simulink model "ProyectoAutomatasSimulink_jona"  (R2015a)
settings: Solver=ode45  SolverMode=SingleTasking  StartTime=0.0  StopTime=inf  FixedStep=dt
values from neighbouring files (symbols this model uses):
  yt0 = 45    [ProyectoAutomatas.m]
libraries: opclib x6, vrlib x1
settings Model: Creator=Garcia Obredor  LastModifiedBy=PIJON 2
settings DataIOCC: SignalLoggingSaveFormat=ModelDataLogs
settings OptimizationCC: BlockReduction=off  BooleanDataType=off  SimCompilerOptimization=on
settings DebuggingCC: SaveWithParameterizedLinksMsg=none  UnderspecifiedInitializationDetection=Classic  MergeDetectMultiDrivingBlocksExec=none  SignalResolutionControl=TryResolveAllWithWarning  MultiTaskDSMMsg=warning  MultiTaskCondExecSysMsg=none
settings HardwareCC: TargetBitPerPointer=64  TargetLongLongMode=on  TargetIntDivRoundTo=Zero  TargetEndianess=LittleEndian  TargetWordSize=64  TargetHWDeviceType=MATLAB Host  ProdEqTarget=off

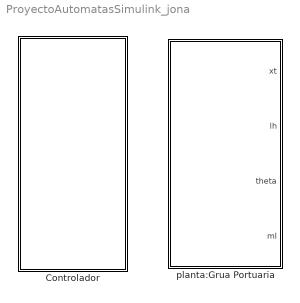
== system ProyectoAutomatasSimulink_jona ==
  Controlador : Subsystem
  planta:Grua Portuaria : Subsystem

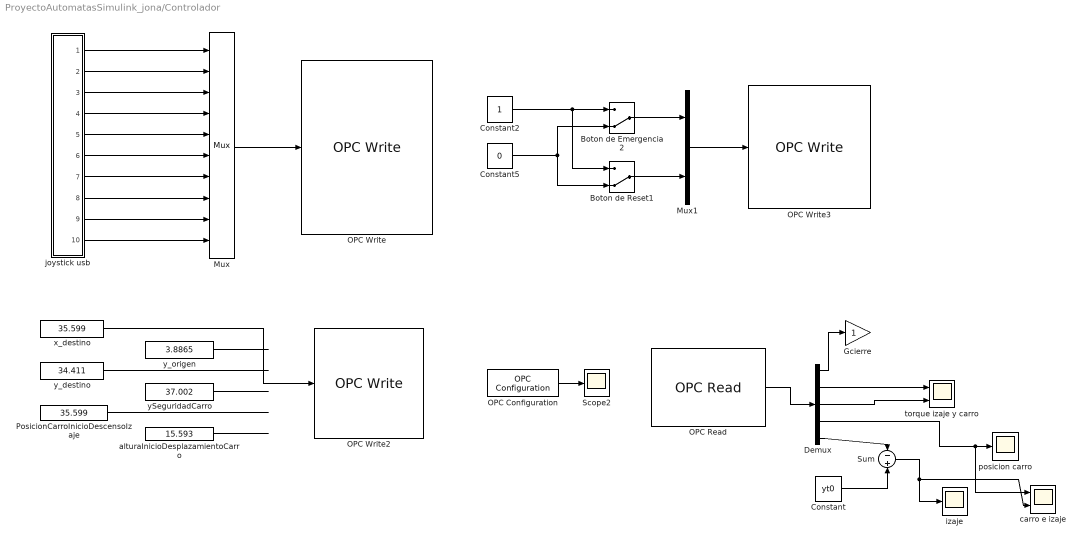
== system ProyectoAutomatasSimulink_jona/Controlador ==
  Boton de Emergencia2 : ManualSwitch  CurrentSetting=0
  Boton de Reset1 : ManualSwitch  CurrentSetting=0
  Constant : Constant  Value=yt0
  Constant2 : Constant
  Constant5 : Constant  Value=0
  Demux : Demux  Outputs=5
  Gcierre : Gain
  Mux : Mux  Inputs=10
  Mux1 : Mux  Inputs=2
  OPC Configuration : opclib/OPC Configuration  opcServers=localhost/CoDeSys.OPC.DA/10  errMissingItems=Error  errReadWrite=Warn  errShutdown=Error  errRTViolation=Warn  rtEnable=on  speedup=1  showLatency=on  beingUsed=on
  OPC Read : opclib/OPC Read  serverHost=localhost  serverID=CoDeSys.OPC.DA  itemIDs=PLC_GW3.Application.Global.Gcierre, PLC_GW3.Application.Global.Th, PLC_GW3.Application.Global.Tt, PLC_GW3.Application.Global.xt, PLC_GW3.Application.Global.lh  readMode=Synchronous (cache)  dataType=double  updateRate=0.001  showQual=off  showTS=off  tsMode=Seconds since start
  OPC Write : opclib/OPC Write  serverHost=localhost  serverID=CoDeSys.OPC.DA  itemIDs=PLC_GW3.Application.Global.BotonAbrirGancho, PLC_GW3.Application.Global.BotonCerrarGancho, PLC_GW3.Application.Global.BotonOperarMaq, PLC_GW3.Application.Global.BotonPararMaq, PLC_GW3.Application.Global.BotonModoAutomatico, PLC_GW3.Application.Global.BotonModoManual, PLC_GW3.Application.Global.PalancaCarro, PLC_GW3.Application.Global.PalancaIzaje, PLC_GW3.Application.Global.BotonActivaControlAngulo, PLC_GW3.Application.Global.BotonDesactivaControlAngulo  writeMode=Synchronous  updateRate=0.001
  OPC Write2 : opclib/OPC Write  serverHost=localhost  serverID=CoDeSys.OPC.DA  itemIDs=PLC_GW3.Application.Global.x_destino  writeMode=Synchronous  updateRate=0.001
  OPC Write3 : opclib/OPC Write  serverHost=localhost  serverID=CoDeSys.OPC.DA  itemIDs=PLC_GW3.Application.Global.BotonEmergencia, PLC_GW3.Application.Global.BotonReset  writeMode=Synchronous  updateRate=0.001
  PosicionCarroInicioDescensoIzaje : Constant  Value=35.599
  Scope2 : Scope
      settings: TimeRange=auto  MaxDataPoints=5000  SaveToWorkspace=off  SaveName=ScopeData  YMin=-0.4375  YMax=3.9375  SampleTime=-1  DataFormat=Array
  Sum : Sum  Inputs=-+
  alturaInicioDesplazamientoCarro : Constant  Value=15.593
  "carro e izaje " : Scope  NumInputPorts=2
      settings: TimeRange=auto  MaxDataPoints=5000  SaveToWorkspace=off  YMin=-150575.73412~-5  YMax=202775.79759~5  SampleTime=-1
  izaje : Scope
      settings: TimeRange=auto  MaxDataPoints=5000  SaveName=posicionIzaje  YMin=1.47924  YMax=22.96427  SampleTime=-1  DataFormat=Array
  joystick usb : Subsystem
  posicion carro : Scope
      settings: TimeRange=auto  MaxDataPoints=5000  SaveName=posicionCarro  YMin=34.91002  YMax=38.94981  SampleTime=-1  DataFormat=Array
  torque izaje y carro : Scope  NumInputPorts=2
      settings: TimeRange=auto  MaxDataPoints=5000  SaveToWorkspace=off  YMin=-150575.73412~-5  YMax=202775.79759~5  SampleTime=-1
  x_destino : Constant  Value=35.599
  ySeguridadCarro : Constant  Value=37.002
  y_destino : Constant  Value=34.411
  y_origen : Constant  Value=3.8865
  wires:
  joystick usb/7(Out8) -> Mux/7
  joystick usb/1(Out1) -> Mux/1
  joystick usb/2(Out2) -> Mux/2
  joystick usb/8(Out9) -> Mux/8
  joystick usb/5(Out6) -> Mux/5
  joystick usb/6(Out7) -> Mux/6
  joystick usb/3(Out3) -> Mux/3
  joystick usb/9(Out5) -> Mux/9
  joystick usb/10(Out10) -> Mux/10
  joystick usb/4(Out4) -> Mux/4
  ySeguridadCarro/1 -> ?
  PosicionCarroInicioDescensoIzaje/1 -> ?
  alturaInicioDesplazamientoCarro/1 -> ?
  y_destino/1 -> ?
  y_origen/1 -> ?
  OPC Configuration/1 -> Scope2/1
  Mux/1 -> OPC Write/1
  x_destino/1 -> OPC Write2/1
  OPC Read/1 -> Demux/1
  Boton de Reset1/1 -> Mux1/2
  Constant5/1 -> Boton de Emergencia2/2, Boton de Reset1/2
  Boton de Emergencia2/1 -> Mux1/1
  Mux1/1 -> OPC Write3/1
  Constant2/1 -> Boton de Emergencia2/1, Boton de Reset1/1
  Demux/1 -> Gcierre/1
  Demux/3 -> torque izaje y carro/2
  Demux/2 -> torque izaje y carro/1
  Demux/4 -> "carro e izaje "/1, posicion carro/1
  Demux/5 -> Sum/1
  Constant/1 -> Sum/2
  Sum/1 -> izaje/1, "carro e izaje "/2

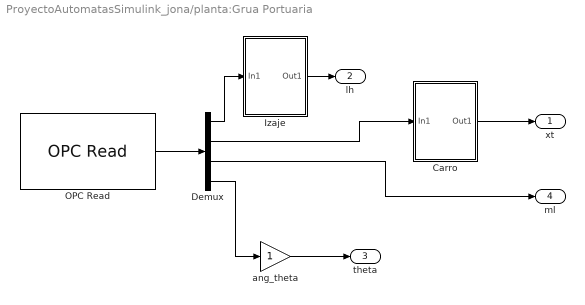
== system ProyectoAutomatasSimulink_jona/planta:Grua Portuaria ==
  Carro : Subsystem
  Demux : Demux
  Izaje : Subsystem
  OPC Read : opclib/OPC Read  serverHost=localhost  serverID=CoDeSys.OPC.DA  itemIDs=PLC_GW3.Application.Global.lh, PLC_GW3.Application.Global.xt, PLC_GW3.Application.Global.ml, PLC_GW3.Application.Global.theta  readMode=Synchronous (cache)  dataType=double  updateRate=0.001  showQual=off  showTS=off  tsMode=Seconds since start
  ang_theta : Gain
  xt : Outport
  lh : Outport  Port=2
  theta : Outport  Port=3
  ml : Outport  Port=4
  wires:
  ang_theta/1 -> theta/1
  OPC Read/1 -> Demux/1
  Demux/4 -> ang_theta/1
  Demux/3 -> ml/1
  Demux/2 -> Carro/1(In1)
  Carro/1(Out1) -> xt/1
  Demux/1 -> Izaje/1(In1)
  Izaje/1(Out1) -> lh/1

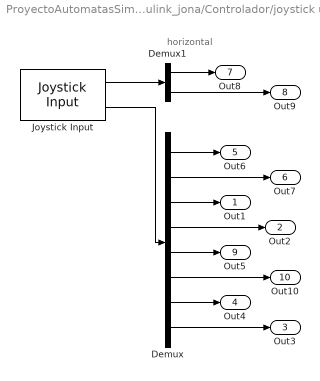
== system ProyectoAutomatasSimulink_jona/Controlador/joystick usb ==
  note: horizontal
  Demux : Demux  Outputs=8
  Demux1 : Demux  Outputs=2
  Joystick Input : vrlib/Joystick Input  joyid=1  adjustports=on  forcefeed=off
  Out1 : Outport
  Out2 : Outport  Port=2
  Out3 : Outport  Port=3
  Out4 : Outport  Port=4
  Out6 : Outport  Port=5
  Out7 : Outport  Port=6
  Out8 : Outport  Port=7
  Out9 : Outport  Port=8
  Out5 : Outport  Port=9
  Out10 : Outport  Port=10
  wires:
  Demux/8 -> Out3/1
  Demux/1 -> Out6/1
  Joystick Input/2 -> Demux/1
  Demux/2 -> Out7/1
  Joystick Input/1 -> Demux1/1
  Demux/7 -> Out4/1
  Demux1/1 -> Out8/1
  Demux1/2 -> Out9/1
  Demux/4 -> Out2/1
  Demux/3 -> Out1/1
  Demux/5 -> Out5/1
  Demux/6 -> Out10/1

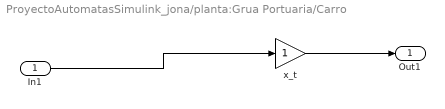
== system ProyectoAutomatasSimulink_jona/planta:Grua Portuaria/Carro ==
  In1 : Inport
  x_t : Gain
  Out1 : Outport
  wires:
  x_t/1 -> Out1/1
  In1/1 -> x_t/1

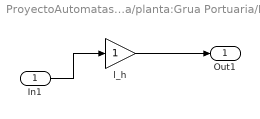
== system ProyectoAutomatasSimulink_jona/planta:Grua Portuaria/Izaje ==
  In1 : Inport
  l_h : Gain
  Out1 : Outport
  wires:
  In1/1 -> l_h/1
  l_h/1 -> Out1/1
